simulink model "Exercise_2"  (R2018a)
settings: Solver=VariableStepAuto  StartTime=0.0  StopTime=1  RelTol=1e-3
libraries: dspsnks4 x2, simulink x2
settings Model: Creator=libingra  LastModifiedBy=libingra

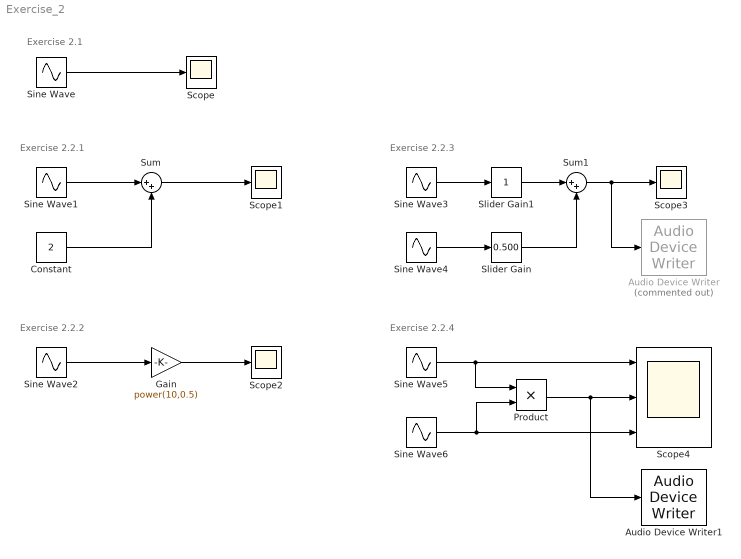
== system Exercise_2 ==
  note: Exercise 2.2.1
  note: Exercise 2.1
  note: Exercise 2.2.2
  note: Exercise 2.2.3
  note: Exercise 2.2.4
  Audio Device Writer : dspsnks4/Audio Device Writer  Commented=on  Driver=ALSA  Device=Default  InheritSampleRate=on  SampleRate=44100  BitDepth=16-bit integer  BufferSize=4096  NumBuffers=10  DefaultOutputChannelMapping=on  OutputChannelMapping=1:2  OutputNumUnderrunSamples=off  DriverIdx=8  DeviceWarnFlag=''
  Audio Device Writer1 : dspsnks4/Audio Device Writer  Driver=ALSA  Device=Default  InheritSampleRate=on  SampleRate=44100  BitDepth=16-bit integer  BufferSize=4096  NumBuffers=10  DefaultOutputChannelMapping=on  OutputChannelMapping=1:2  OutputNumUnderrunSamples=off  DriverIdx=8  DeviceWarnFlag=''
  Constant : Constant  Value=2
  Gain : Gain  Gain=power(10,0.5)
  Product : Product
  Scope{,1..3} (4 alike) : Scope
  Scope4 : Scope  NumInputPorts=3
  Sine Wave{,1..3} (4 alike) : Sin  SineType=Sample based  Frequency=2*pi*2  Samples=48  SampleTime=1/48000
  Sine Wave4 : Sin  SineType=Sample based  Samples=24  SampleTime=1/48000
  Sine Wave5 : Sin  SineType=Sample based  Frequency=2*pi*31.25  Samples=96  SampleTime=1/48000
  Sine Wave6 : Sin  SineType=Sample based  Frequency=2*pi*500  Samples=1536  SampleTime=1/48000
  Slider Gain : simulink/Math Operations/Slider Gain  gain=0.500  low=0  high=1
  Slider Gain1 : simulink/Math Operations/Slider Gain  gain=1  low=0  high=2
  Sum : Sum  Inputs=|++
  Sum1 : Sum  Inputs=|++
  wires:
  Sine Wave/1 -> Scope/1
  Constant/1 -> Sum/2
  Sine Wave1/1 -> Sum/1
  Sum/1 -> Scope1/1
  Sine Wave2/1 -> Gain/1
  Gain/1 -> Scope2/1
  Sum1/1 -> Scope3/1, Audio Device Writer/1
  Sine Wave3/1 -> Slider Gain1/1
  Slider Gain1/1 -> Sum1/1
  Sine Wave4/1 -> Slider Gain/1
  Slider Gain/1 -> Sum1/2
  Sine Wave6/1 -> Product/2, Scope4/3
  Product/1 -> Audio Device Writer1/1, Scope4/2
  Sine Wave5/1 -> Product/1, Scope4/1
